simulink subsystem "ConfiguredSimulinkPlantModels"  (R2022b)
settings: Solver=VariableStepAuto  StartTime=0.0  StopTime=10.0  RelTol=1e-3
undefined symbols (not defined in the file): OCV, OCV_SoC, PlntTrnsfrCaseAxlSpdLock, PlntTrnsfrCaseTrqSplitRatio, soc_init
settings Model: Creator=The MathWorks, Inc.  LastModifiedBy=Thomas

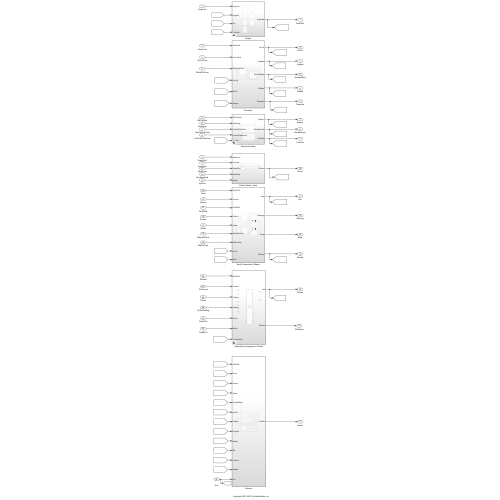
[thumbnail: Simulink's stored preview of the top-level diagram]
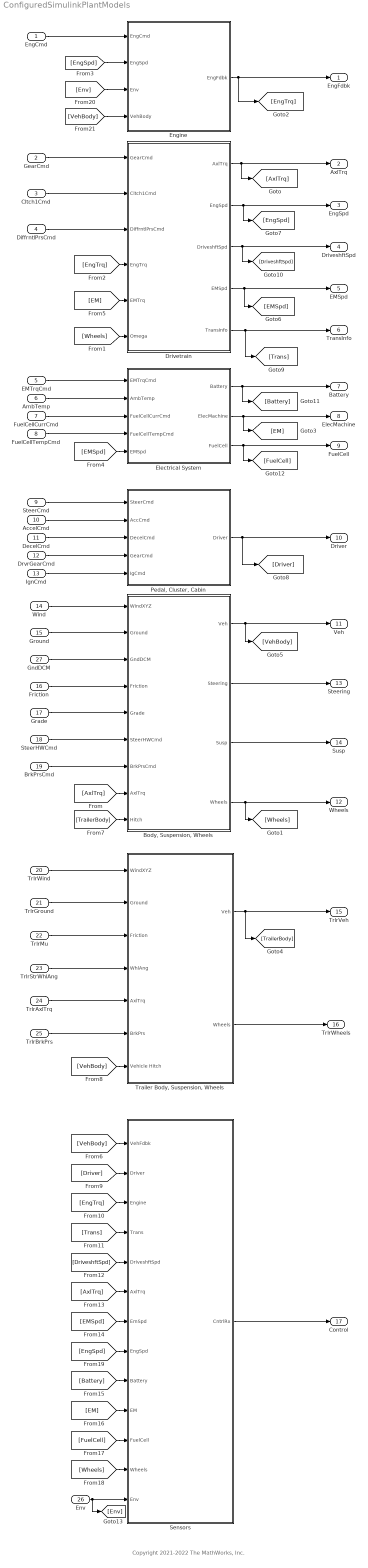
== system ConfiguredSimulinkPlantModels ==
  note: Copyright 2021-2022 The MathWorks, Inc.
  EngCmd : Inport
  GearCmd : Inport  Port=2
  Cltch1Cmd : Inport  Port=3
  DiffrntlPrsCmd : Inport  Port=4
  EMTrqCmd : Inport  Port=5
  AmbTemp : Inport  Port=6
  FuelCellCurrCmd : Inport  Port=7
  FuelCellTempCmd : Inport  Port=8
  SteerCmd : Inport  Port=9
  AccelCmd : Inport  Port=10
  DecelCmd : Inport  Port=11
  DrvrGearCmd : Inport  Port=12
  IgnCmd : Inport  Port=13
  Wind : Inport  Port=14
  Ground : Inport  Port=15
  Friction : Inport  Port=16
  Grade : Inport  Port=17
  SteerHWCmd : Inport  Port=18
  BrkPrsCmd : Inport  Port=19
  TrlrWind : Inport  Port=20
  TrlrGround : Inport  Port=21
  TrlrMu : Inport  Port=22
  TrlrStrWhlAng : Inport  Port=23
  TrlrAxlTrq : Inport  Port=24
  TrlrBrkPrs : Inport  Port=25
  " Env" : Inport  Port=26
  GndDCM : Inport  Port=27
  "Body, Suspension, Wheels" : Subsystem  VariantControl=Lateral Vehicle Dynamics
  Drivetrain : Subsystem
  Electrical System : Subsystem  Variant=on  VariantControlMode=label  VariantControl=Choice  LabelModeActiveChoice=Electrical System 1EM
  Engine : Subsystem  Variant=on  VariantControlMode=label  LabelModeActiveChoice=No Engine
  "Pedal, Cluster, Cabin" : Subsystem
  Sensors : Subsystem
  "Trailer Body, Suspension, Wheels" : Subsystem  Variant=on  VariantControlMode=label  LabelModeActiveChoice=No Trailer
  EngFdbk : Outport
  AxlTrq : Outport  Port=2
  EngSpd : Outport  Port=3
  DriveshftSpd : Outport  Port=4
  EMSpd : Outport  Port=5
  TransInfo : Outport  Port=6
  Battery : Outport  Port=7
  ElecMachine : Outport  Port=8
  FuelCell : Outport  Port=9
  Driver : Outport  Port=10
  Veh : Outport  Port=11
  Wheels : Outport  Port=12
  Steering : Outport  Port=13
  Susp : Outport  Port=14
  TrlrVeh : Outport  Port=15
  TrlrWheels : Outport  Port=16
  Control : Outport  Port=17
  wires:
  [EngSpd] -> Sensors/8(EngSpd)
  Cltch1Cmd/1 -> Drivetrain/2(Cltch1Cmd)
  FuelCellTempCmd/1 -> Electrical System/4(FuelCellTempCmd)
  "Body, Suspension, Wheels"/1(Veh) -> Veh/1, [VehBody]
  Electrical System/3(FuelCell) -> FuelCell/1, [FuelCell]
  [EngSpd] -> Engine/2(EngSpd)
  "Body, Suspension, Wheels"/3(Susp) -> Susp/1
  Grade/1 -> "Body, Suspension, Wheels"/5(Grade)
  [VehBody] -> Sensors/1(VehFdbk)
  SteerHWCmd/1 -> "Body, Suspension, Wheels"/6(SteerHWCmd)
  "Pedal, Cluster, Cabin"/1(Driver) -> Driver/1, [Driver]
  " Env"/1 -> Sensors/13(Env), [Env]
  [Driver] -> Sensors/2(Driver)
  AccelCmd/1 -> "Pedal, Cluster, Cabin"/2(AccCmd)
  [VehBody] -> Engine/4(VehBody)
  Drivetrain/3(DriveshftSpd) -> DriveshftSpd/1, [DriveshftSpd]
  [Wheels] -> Drivetrain/6(Omega)
  [EngTrq] -> Drivetrain/4(EngTrq)
  [Env] -> Engine/3(Env)
  IgnCmd/1 -> "Pedal, Cluster, Cabin"/5(IgCmd)
  TrlrGround/1 -> "Trailer Body, Suspension, Wheels"/2(Ground)
  [Battery] -> Sensors/9(Battery)
  [FuelCell] -> Sensors/11(FuelCell)
  [EM] -> Sensors/10(EM)
  [DriveshftSpd] -> Sensors/5(DriveshftSpd)
  [AxlTrq] -> Sensors/6(AxlTrq)
  DecelCmd/1 -> "Pedal, Cluster, Cabin"/3(DecelCmd)
  Drivetrain/4(EMSpd) -> EMSpd/1, [EMSpd]
  "Body, Suspension, Wheels"/4(Wheels) -> [Wheels], Wheels/1
  GearCmd/1 -> Drivetrain/1(GearCmd)
  SteerCmd/1 -> "Pedal, Cluster, Cabin"/1(SteerCmd)
  DrvrGearCmd/1 -> "Pedal, Cluster, Cabin"/4(GearCmd)
  [VehBody] -> "Trailer Body, Suspension, Wheels"/7(Vehicle Hitch)
  Friction/1 -> "Body, Suspension, Wheels"/4(Friction)
  EMTrqCmd/1 -> Electrical System/1(EMTrqCmd)
  GndDCM/1 -> "Body, Suspension, Wheels"/3(GndDCM)
  Sensors/1(CntrlRx) -> Control/1
  [EngTrq] -> Sensors/3(Engine)
  Electrical System/2(ElecMachine) -> ElecMachine/1, [EM]
  Drivetrain/2(EngSpd) -> EngSpd/1, [EngSpd]
  [Trans] -> Sensors/4(Trans)
  Wind/1 -> "Body, Suspension, Wheels"/1(WindXYZ)
  "Trailer Body, Suspension, Wheels"/1(Veh) -> TrlrVeh/1, [TrailerBody]
  TrlrBrkPrs/1 -> "Trailer Body, Suspension, Wheels"/6(BrkPrs)
  TrlrWind/1 -> "Trailer Body, Suspension, Wheels"/1(WindXYZ)
  DiffrntlPrsCmd/1 -> Drivetrain/3(DiffrntlPrsCmd)
  Drivetrain/1(AxlTrq) -> AxlTrq/1, [AxlTrq]
  BrkPrsCmd/1 -> "Body, Suspension, Wheels"/7(BrkPrsCmd)
  TrlrStrWhlAng/1 -> "Trailer Body, Suspension, Wheels"/4(WhlAng)
  TrlrMu/1 -> "Trailer Body, Suspension, Wheels"/3(Friction)
  EngCmd/1 -> Engine/1(EngCmd)
  [EM] -> Drivetrain/5(EMTrq)
  "Body, Suspension, Wheels"/2(Steering) -> Steering/1
  Engine/1(EngFdbk) -> EngFdbk/1, [EngTrq]
  Ground/1 -> "Body, Suspension, Wheels"/2(Ground)
  TrlrAxlTrq/1 -> "Trailer Body, Suspension, Wheels"/5(AxlTrq)
  [AxlTrq] -> "Body, Suspension, Wheels"/8(AxlTrq)
  [TrailerBody] -> "Body, Suspension, Wheels"/9(Hitch)
  AmbTemp/1 -> Electrical System/2(AmbTemp)
  Drivetrain/5(TransInfo) -> TransInfo/1, [Trans]
  Electrical System/1(Battery) -> Battery/1, [Battery]
  "Trailer Body, Suspension, Wheels"/2(Wheels) -> TrlrWheels/1
  [Wheels] -> Sensors/12(Wheels)
  [EMSpd] -> Sensors/7(EmSpd)
  FuelCellCurrCmd/1 -> Electrical System/3(FuelCellCurrCmd)
  [EMSpd] -> Electrical System/5(EMSpd)

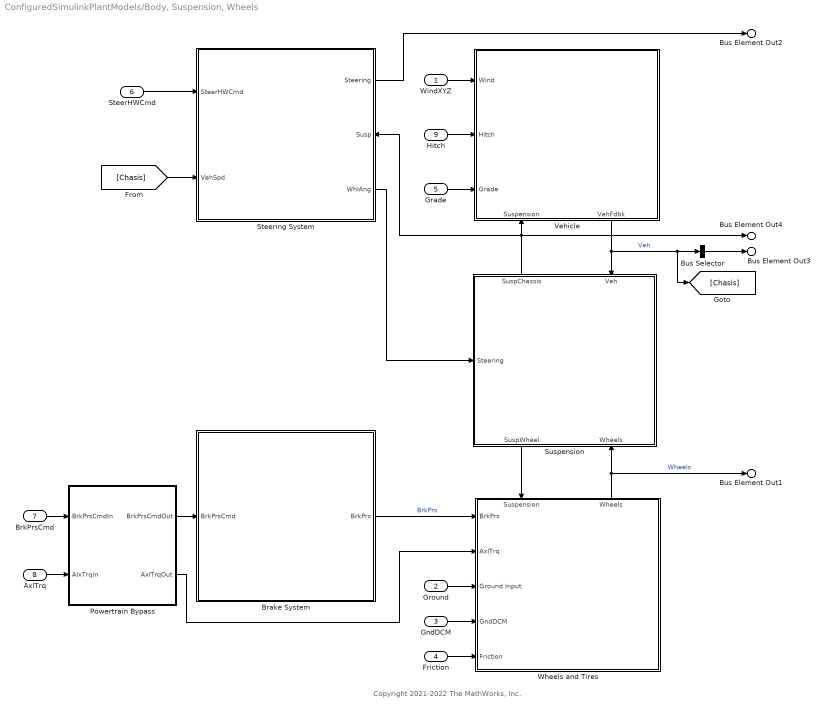
== system ConfiguredSimulinkPlantModels/Body, Suspension, Wheels ==
  note: Copyright 2021-2022 The MathWorks, Inc.
  WindXYZ : Inport  Unit=m/s  PortDimensions=3
  Ground : Inport  Port=2  Unit=m  PortDimensions=4
  GndDCM : Inport  Port=3
  Friction : Inport  Port=4  Unit=1  PortDimensions=4
  Grade : Inport  Port=5
  SteerHWCmd : Inport  Port=6  Unit=rad
  BrkPrsCmd : Inport  Port=7  PortDimensions=4
  AxlTrq : Inport  Port=8  Unit=N*m  PortDimensions=4
  Hitch : Inport  Port=9
  Brake System : Subsystem  Variant=on  VariantControlMode=label  VariantControl=Choice  LabelModeActiveChoice=BrakingHydraulics
      mask Display: disp('Brake System');
  Bus Selector : BusSelector  OutputSignals=InertFrm,BdyFrm  OutputAsBus=on
  Powertrain Bypass : Subsystem  Variant=on  VariantControlMode=label  VariantControl=Choice  LabelModeActiveChoice=Pass Through
  Steering System : Subsystem  Variant=on  VariantControlMode=label  VariantControl=0  LabelModeActiveChoice=No Steering
      settings: PortSchema="{\"entries\":[{\"content\":{\"sides\":[{\"content\":{\"connectorIds\":[\"In1\",\"In2\"]},\"type\":\"ConnectorPlacement.EquallySpacedRectSide\",\"uuid\":\"f4eae9a1-ee72-4894-9c3f-d81ee40fba89\"},{\"content\":{\"connectorIds\":[\"Out1\",\"In3\",\"Out2\"],\"side\":\"RIGHT\"},\"type\":\"ConnectorPlacement.EquallySpacedRectSide\",\"uuid\":\"c62a78d9-dc5d-4f96-a554-c82d7fa22a9e\"},{\"content\":{\"connectorIds\":[],\"side\":\"TOP\"},\"type\":\"ConnectorPlacement.EquallySpacedRectSide\",\"uuid\":\"38f3851a-1d1e-4a2b-8c09-8e5c8dcc7723\"}]},\"type\":\"ConnectorPlacement.EquallySpacedConnector\",\"uuid\":\"9f269846-92fa-4948-bc2b-71154f41fdde\"}],\"packageUris\":[\"http://schema.mathworks.com/mf0/Connector/R2020b\"],\"version\":\"1.0\"}"
      mask Display: disp('Steering System');
  Suspension : Subsystem  Variant=on  VariantControlMode=label  VariantControl=Choice  LabelModeActiveChoice=No Suspension
      settings: PortSchema="{\"entries\":[{\"content\":{\"sides\":[{\"content\":{\"connectorIds\":[\"In1\"]},\"type\":\"ConnectorPlacement.EquallySpacedRectSide\",\"uuid\":\"0a9265e3-f55e-4b74-9b74-681dc9522591\"},{\"content\":{\"connectorIds\":[],\"side\":\"RIGHT\"},\"type\":\"ConnectorPlacement.EquallySpacedRectSide\",\"uuid\":\"92df639a-7bc2-4e90-97ea-0cb216e2f16a\"},{\"content\":{\"connectorIds\":[\"Out2\",\"In2\"],\"side\":\"TOP\"},\"type\":\"ConnectorPlacement.EquallySpacedRectSide\",\"uuid\":\"2064b6cb-c7a8-4cfb-82de-a07750d990cb\"},{\"content\":{\"connectorIds\":[\"Out1\",\"In3\"],\"side\":\"BOTTOM\"},\"type\":\"ConnectorPlacement.EquallySpacedRectSide\",\"uuid\":\"169bd4e6-c3fe-4e36-acea-c25875014463\"}]},\"type\":\"ConnectorPlacement.EquallySpacedConnector\",\"uuid\":\"e0b50182-0637-4594-80e7-4ddd0df85797\"}],\"packageUris\":[\"http://schema.mathworks.com/mf0/Connector/R2020b\"],\"version\":\"1.0\"}"
      mask Display: disp('Suspension');
  Vehicle : Subsystem  Variant=on  VariantControlMode=label  VariantControl=Choice  LabelModeActiveChoice=Vehicle Body 3DOF Longitudinal
      settings: PortSchema="{\"entries\":[{\"content\":{\"sides\":[{\"content\":{\"connectorIds\":[\"In1\",\"In2\",\"In3\"]},\"type\":\"ConnectorPlacement.EquallySpacedRectSide\",\"uuid\":\"0a9265e3-f55e-4b74-9b74-681dc9522591\"},{\"content\":{\"connectorIds\":[],\"side\":\"RIGHT\"},\"type\":\"ConnectorPlacement.EquallySpacedRectSide\",\"uuid\":\"92df639a-7bc2-4e90-97ea-0cb216e2f16a\"},{\"content\":{\"connectorIds\":[],\"side\":\"TOP\"},\"type\":\"ConnectorPlacement.EquallySpacedRectSide\",\"uuid\":\"2064b6cb-c7a8-4cfb-82de-a07750d990cb\"},{\"content\":{\"connectorIds\":[\"In4\",\"Out1\"],\"side\":\"BOTTOM\"},\"type\":\"ConnectorPlacement.EquallySpacedRectSide\",\"uuid\":\"2b34afca-0a88-43db-924f-6476183b84bd\"}]},\"type\":\"ConnectorPlacement.EquallySpacedConnector\",\"uuid\":\"e0b50182-0637-4594-80e7-4ddd0df85797\"}],\"packageUris\":[\"http://schema.mathworks.com/mf0/Connector/R2020b\"],\"version\":\"1.0\"}"
      mask Display: disp('Vehicle');
  Wheels and Tires : Subsystem  Variant=on  VariantControlMode=label  VariantControl=Choice  LabelModeActiveChoice=MF Tires Longitudinal
      settings: PortSchema="{\"entries\":[{\"content\":{\"sides\":[{\"content\":{\"connectorIds\":[\"In1\",\"In2\",\"In3\",\"In4\",\"In5\"]},\"type\":\"ConnectorPlacement.EquallySpacedRectSide\",\"uuid\":\"fdb4d4cd-d0c0-42d9-b073-775af31e96a1\"},{\"content\":{\"connectorIds\":[],\"side\":\"RIGHT\"},\"type\":\"ConnectorPlacement.EquallySpacedRectSide\",\"uuid\":\"04106ddf-9917-4cd4-b177-ae763d642686\"},{\"content\":{\"connectorIds\":[\"In6\",\"Out1\"],\"side\":\"TOP\"},\"type\":\"ConnectorPlacement.EquallySpacedRectSide\",\"uuid\":\"568bf95c-0e25-4c45-a134-c198357b75be\"}]},\"type\":\"ConnectorPlacement.EquallySpacedConnector\",\"uuid\":\"4f44df5e-0d14-43ea-934e-2abe86546e95\"}],\"packageUris\":[\"http://schema.mathworks.com/mf0/Connector/R2020b\"],\"version\":\"1.0\"}"
      mask Display: disp('Wheels and Tires');
  Bus Element Out3 : Outport  PortName=Veh
  Bus Element Out2 : Outport  Port=2  PortName=Steering
  Bus Element Out4 : Outport  Port=3  PortName=Susp
  Bus Element Out1 : Outport  Port=4  PortName=Wheels
  wires:
  GndDCM/1 -> Wheels and Tires/4(GndDCM)
  Friction/1 -> Wheels and Tires/5(Friction)
  Powertrain Bypass/2(AxlTrqOut) -> Wheels and Tires/2(AxlTrq)
  Ground/1 -> Wheels and Tires/3(Ground Input)
  Grade/1 -> Vehicle/3(Grade)
  Wheels and Tires/1(Wheels) -> Suspension/3(Wheels), Bus Element Out1/1  "Wheels"
  Suspension/1(SuspWheel) -> Wheels and Tires/6(Suspension)
  Brake System/1(BrkPrs) -> Wheels and Tires/1(BrkPrs)  "BrkPrs"
  Vehicle/1(VehFdbk) -> Suspension/2(Veh), [Chasis], Bus Selector/1  "Veh"
  Hitch/1 -> Vehicle/2(Hitch)
  WindXYZ/1 -> Vehicle/1(Wind)
  Suspension/2(SuspChassis) -> Bus Element Out4/1, Vehicle/4(Suspension), Steering System/3(Susp)
  Steering System/2(WhlAng) -> Suspension/1(Steering)
  BrkPrsCmd/1 -> Powertrain Bypass/1(BrkPrsCmdIn)
  Bus Selector/1 -> Bus Element Out3/1
  [Chasis] -> Steering System/2(VehSpd)
  SteerHWCmd/1 -> Steering System/1(SteerHWCmd)
  Steering System/1(Steering) -> Bus Element Out2/1
  Powertrain Bypass/1(BrkPrsCmdOut) -> Brake System/1(BrkPrsCmd)
  AxlTrq/1 -> Powertrain Bypass/2(AlxTrqIn)

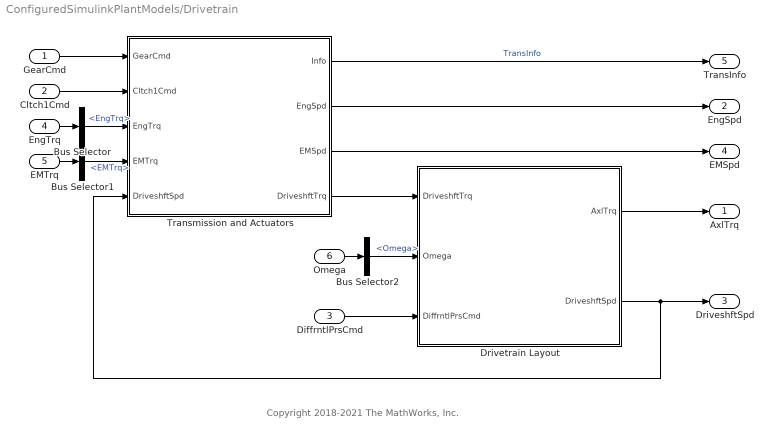
== system ConfiguredSimulinkPlantModels/Drivetrain ==
  note: Copyright 2018-2021 The MathWorks, Inc.
  GearCmd : Inport
  Cltch1Cmd : Inport  Port=2
  DiffrntlPrsCmd : Inport  Port=3
  EngTrq : Inport  Port=4
  EMTrq : Inport  Port=5
  Omega : Inport  Port=6
  Bus Selector : BusSelector  OutputSignals=EngTrq
  Bus Selector1 : BusSelector  OutputSignals=EMTrq
  Bus Selector2 : BusSelector  OutputSignals=Wheels.Omega
  Drivetrain Layout : Subsystem  VariantControl=New
  Transmission and Actuators : Subsystem  Variant=on  VariantControlMode=label  LabelModeActiveChoice=Electric Vehicle 1EM
  AxlTrq : Outport  VectorParamsAs1DForOutWhenUnconnected=off
  EngSpd : Outport  Port=2  Unit=rad/s  VectorParamsAs1DForOutWhenUnconnected=off
  DriveshftSpd : Outport  Port=3  VectorParamsAs1DForOutWhenUnconnected=off
  EMSpd : Outport  Port=4  Unit=rad/s  VectorParamsAs1DForOutWhenUnconnected=off
  TransInfo : Outport  Port=5  VectorParamsAs1DForOutWhenUnconnected=off
  wires:
  Transmission and Actuators/1(Info) -> TransInfo/1  "TransInfo"
  DiffrntlPrsCmd/1 -> Drivetrain Layout/3(DiffrntlPrsCmd)
  Cltch1Cmd/1 -> Transmission and Actuators/2(Cltch1Cmd)
  Drivetrain Layout/2(DriveshftSpd) -> DriveshftSpd/1, Transmission and Actuators/5(DriveshftSpd)
  GearCmd/1 -> Transmission and Actuators/1(GearCmd)
  Drivetrain Layout/1(AxlTrq) -> AxlTrq/1
  Transmission and Actuators/2(EngSpd) -> EngSpd/1
  Transmission and Actuators/3(EMSpd) -> EMSpd/1
  Transmission and Actuators/4(DriveshftTrq) -> Drivetrain Layout/1(DriveshftTrq)
  EngTrq/1 -> Bus Selector/1
  Bus Selector/1 -> Transmission and Actuators/3(EngTrq)  "<EngTrq>"
  EMTrq/1 -> Bus Selector1/1
  Bus Selector1/1 -> Transmission and Actuators/4(EMTrq)  "<EMTrq>"
  Omega/1 -> Bus Selector2/1
  Bus Selector2/1 -> Drivetrain Layout/2(Omega)  "<Omega>"

== system ConfiguredSimulinkPlantModels/Electrical System ==
  EMTrqCmd : Inport
  AmbTemp : Inport  Port=2
  FuelCellCurrCmd : Inport  Port=3
  FuelCellTempCmd : Inport  Port=4
  EMSpd : Inport  Port=5
  Electrical System 1EM : Subsystem  VariantControl=Electrical System 1EM
  Battery : Outport
  ElecMachine : Outport  Port=2
  FuelCell : Outport  Port=3

== system ConfiguredSimulinkPlantModels/Engine ==
  EngCmd : Inport
  EngSpd : Inport  Port=2
  Env : Inport  Port=3
  VehBody : Inport  Port=4
  No Engine : Subsystem  VariantControl=No Engine
  EngFdbk : Outport  VectorParamsAs1DForOutWhenUnconnected=off

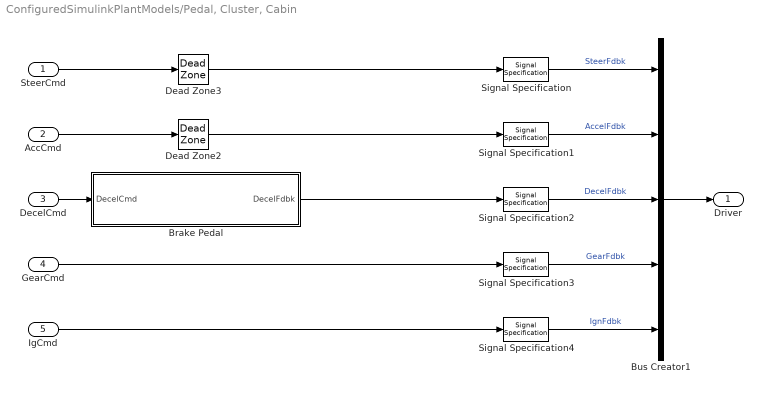
== system ConfiguredSimulinkPlantModels/Pedal, Cluster, Cabin ==
  SteerCmd : Inport
  AccCmd : Inport  Port=2
  DecelCmd : Inport  Port=3
  GearCmd : Inport  Port=4
  IgCmd : Inport  Port=5
  Brake Pedal : Subsystem
  Bus Creator1 : BusCreator  Inputs=5
  Dead Zone2 : DeadZone  LowerValue=0  UpperValue=.01  ZeroCross=off
  Dead Zone3 : DeadZone  LowerValue=-.01  UpperValue=.01  ZeroCross=off
  Signal Specification : SignalSpecification  Unit=rad
  Signal Specification{1..4} (4 alike) : SignalSpecification  Unit=1
  Driver : Outport
  wires:
  Dead Zone3/1 -> Signal Specification/1
  Signal Specification1/1 -> Bus Creator1/2  "AccelFdbk"
  Signal Specification4/1 -> Bus Creator1/5  "IgnFdbk"
  Brake Pedal/1(DecelFdbk) -> Signal Specification2/1
  Signal Specification/1 -> Bus Creator1/1  "SteerFdbk"
  Signal Specification2/1 -> Bus Creator1/3  "DecelFdbk"
  GearCmd/1 -> Signal Specification3/1
  Bus Creator1/1 -> Driver/1
  IgCmd/1 -> Signal Specification4/1
  Signal Specification3/1 -> Bus Creator1/4  "GearFdbk"
  Dead Zone2/1 -> Signal Specification1/1
  SteerCmd/1 -> Dead Zone3/1
  AccCmd/1 -> Dead Zone2/1
  DecelCmd/1 -> Brake Pedal/1(DecelCmd)

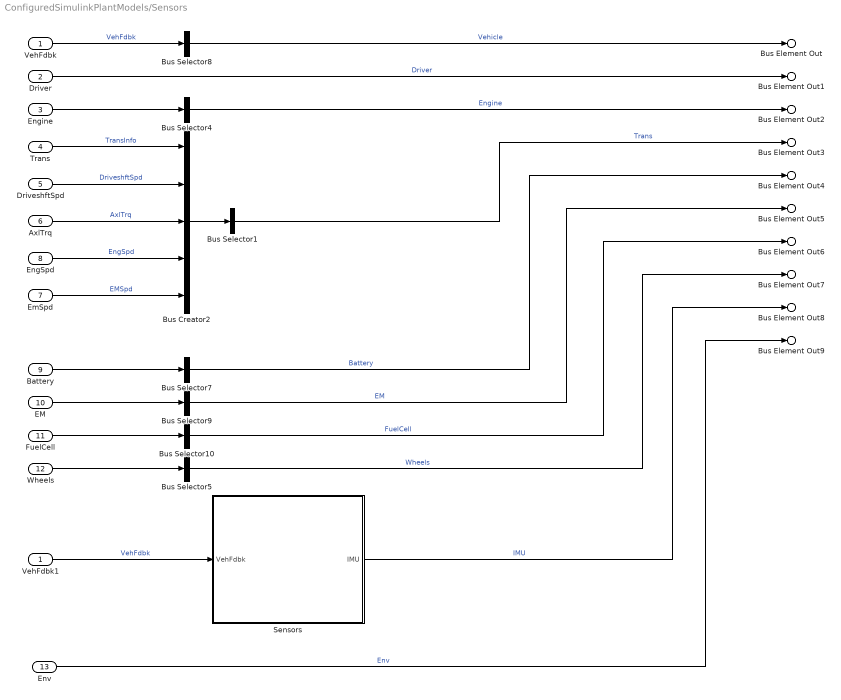
== system ConfiguredSimulinkPlantModels/Sensors ==
  VehFdbk : Inport
  Driver : Inport  Port=2
  Engine : Inport  Port=3
  Trans : Inport  Port=4
  DriveshftSpd : Inport  Port=5
  AxlTrq : Inport  Port=6
  EmSpd : Inport  Port=7
  EngSpd : Inport  Port=8
  Battery : Inport  Port=9
  EM : Inport  Port=10
  FuelCell : Inport  Port=11
  Wheels : Inport  Port=12
  Env : Inport  Port=13
  Bus Creator2 : BusCreator  Inputs=5
  Bus Selector1 : BusSelector  OutputSignals=TransInfo.Cltch1State,TransInfo.Cltch2State,DriveshftSpd,AxlTrq,EngSpd,EMSpd,TransInfo.TransInfo.Trans.TransGear  OutputAsBus=on
  Bus Selector10 : BusSelector  OutputSignals=FuelCellVolt,FuelCellCurr,H2Flw  OutputAsBus=on
  Bus Selector4 : BusSelector  OutputSignals=EngTrq,Map,Mat,ThrPosPct,WgAreaPct,IntkCamPhase,ExhCamPhase,TurboRackPos,EgrVlvAreaPct,VarCompRatioPos,IntkVlvLift,VarIntkRunLen,Afr,IntkSwirlVlvPos,TurboSpd,Iat,Ect,EgrVlvDeltaPrs,EgrVlvInTemp  OutputAsBus=on
  Bus Selector5 : BusSelector  OutputSignals=Wheels.BrkPrs,Wheels.Kappa,Wheels.Alpha,Wheels.Omega  OutputAsBus=on
  Bus Selector7 : BusSelector  OutputSignals=BattSoc,BattVolt,BattCurr,BattPwr,BMSSensors  OutputAsBus=on
  Bus Selector8 : BusSelector  OutputSignals=BdyFrm.Cg.Vel.xdot  OutputAsBus=on
  Bus Selector9 : BusSelector  OutputSignals=EMTrq,EMPwrElec  OutputAsBus=on
  Sensors : Subsystem  Variant=on  VariantControlMode=label  VariantControl=Choice  LabelModeActiveChoice=No IMU Sensor
  VehFdbk1 : InportShadow
  Bus Element Out : Outport  PortName=CntrlRx  Element=Vehicle
  Bus Element Out1 : Outport  PortName=CntrlRx  Element=Driver
  Bus Element Out2 : Outport  PortName=CntrlRx  Element=Engine
  Bus Element Out3 : Outport  PortName=CntrlRx  Element=Trans
  Bus Element Out4 : Outport  PortName=CntrlRx  Element=Battery
  Bus Element Out5 : Outport  PortName=CntrlRx  Element=EM
  Bus Element Out6 : Outport  PortName=CntrlRx  Element=FuelCell
  Bus Element Out7 : Outport  PortName=CntrlRx  Element=Wheels
  Bus Element Out8 : Outport  PortName=CntrlRx  Element=IMU
  Bus Element Out9 : Outport  PortName=CntrlRx  Element=Env
  wires:
  Bus Selector1/1 -> Bus Element Out3/1  "Trans"
  Bus Creator2/1 -> Bus Selector1/1
  Trans/1 -> Bus Creator2/1  "TransInfo"
  EngSpd/1 -> Bus Creator2/4  "EngSpd"
  Env/1 -> Bus Element Out9/1  "Env"
  Driver/1 -> Bus Element Out1/1  "Driver"
  Sensors/1(IMU) -> Bus Element Out8/1  "IMU"
  VehFdbk1/1 -> Sensors/1(VehFdbk)  "VehFdbk"
  Wheels/1 -> Bus Selector5/1
  FuelCell/1 -> Bus Selector10/1
  EM/1 -> Bus Selector9/1
  Battery/1 -> Bus Selector7/1
  EmSpd/1 -> Bus Creator2/5  "EMSpd"
  AxlTrq/1 -> Bus Creator2/3  "AxlTrq"
  DriveshftSpd/1 -> Bus Creator2/2  "DriveshftSpd"
  Engine/1 -> Bus Selector4/1
  VehFdbk/1 -> Bus Selector8/1  "VehFdbk"
  Bus Selector4/1 -> Bus Element Out2/1  "Engine"
  Bus Selector10/1 -> Bus Element Out6/1  "FuelCell"
  Bus Selector9/1 -> Bus Element Out5/1  "EM"
  Bus Selector8/1 -> Bus Element Out/1  "Vehicle"
  Bus Selector7/1 -> Bus Element Out4/1  "Battery"
  Bus Selector5/1 -> Bus Element Out7/1  "Wheels"

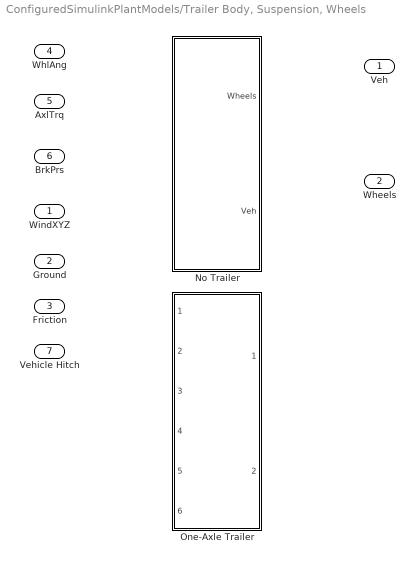
== system ConfiguredSimulinkPlantModels/Trailer Body, Suspension, Wheels ==
  WindXYZ : Inport
  Ground : Inport  Port=2
  Friction : Inport  Port=3
  WhlAng : Inport  Port=4
  AxlTrq : Inport  Port=5
  BrkPrs : Inport  Port=6
  Vehicle Hitch : Inport  Port=7
  No Trailer : Subsystem  VariantControl=No Trailer
  One-Axle Trailer : Subsystem  VariantControl=One-Axle Trailer  ReferencedSubsystem=OneAxleTrailer
  Veh : Outport  VectorParamsAs1DForOutWhenUnconnected=off
  Wheels : Outport  Port=2  VectorParamsAs1DForOutWhenUnconnected=off

== system ConfiguredSimulinkPlantModels/Body, Suspension, Wheels/Brake System ==
  BrkPrsCmd : Inport
  BrakingHydraulics : Subsystem  VariantControl=BrakingHydraulics  ReferencedSubsystem=BrakingHydraulics
  BrkPrs : Outport

== system ConfiguredSimulinkPlantModels/Body, Suspension, Wheels/Powertrain Bypass ==
  BrkPrsCmdIn : Inport
  AlxTrqIn : Inport  Port=2
  External Signal Source : Subsystem  VariantControl=External Signal Source
  Pass Through : Subsystem  VariantControl=Pass Through
  BrkPrsCmdOut : Outport
  AxlTrqOut : Outport  Port=2

== system ConfiguredSimulinkPlantModels/Body, Suspension, Wheels/Steering System ==
  SteerHWCmd : Inport
  VehSpd : Inport  Port=2
  Susp : Inport  Port=3
  No Steering : Subsystem  VariantControl=No Steering  ReferencedSubsystem=NoSteering
  Steering : Outport
  WhlAng : Outport  Port=2  VectorParamsAs1DForOutWhenUnconnected=off

== system ConfiguredSimulinkPlantModels/Body, Suspension, Wheels/Suspension ==
  Steering : Inport
  Veh : Inport  Port=2
  Wheels : Inport  Port=3
  No Suspension : Subsystem  VariantControl=No Suspension  ReferencedSubsystem=NoSuspension
  SuspWheel : Outport
  SuspChassis : Outport  Port=2

== system ConfiguredSimulinkPlantModels/Body, Suspension, Wheels/Vehicle ==
  Wind : Inport
  Hitch : Inport  Port=2
  Grade : Inport  Port=3
  Suspension : Inport  Port=4
  Vehicle Body 3DOF Longitudinal : Subsystem  VariantControl=Vehicle Body 3DOF Longitudinal  ReferencedSubsystem=VehicleBody3DOFLongitudinal
  VehFdbk : Outport

== system ConfiguredSimulinkPlantModels/Body, Suspension, Wheels/Wheels and Tires ==
  BrkPrs : Inport
  AxlTrq : Inport  Port=2
  Ground Input : Inport  Port=3
  GndDCM : Inport  Port=4
  Friction : Inport  Port=5
  Suspension : Inport  Port=6
  MF Tires Longitudinal : Subsystem  VariantControl=MF Tires Longitudinal  ReferencedSubsystem=MFTiresLongitudinal
  Wheels : Outport

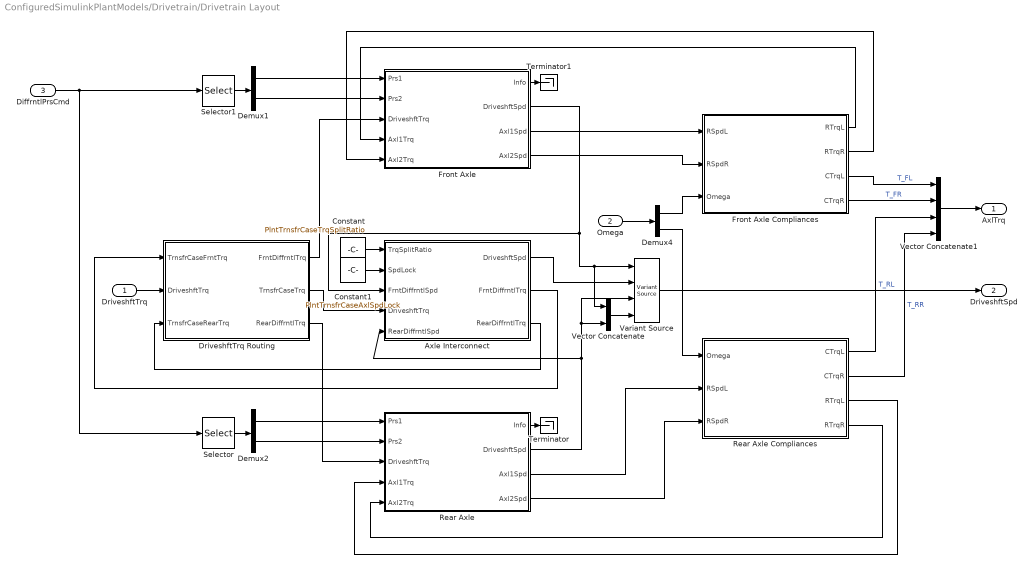
== system ConfiguredSimulinkPlantModels/Drivetrain/Drivetrain Layout ==
  DriveshftTrq : Inport
  Omega : Inport  Port=2
  DiffrntlPrsCmd : Inport  Port=3
  Axle Interconnect : Subsystem  Variant=on  VariantControlMode=label  VariantControl=Choice  LabelModeActiveChoice=No Interconnect
  Constant : Constant  Value=PlntTrnsfrCaseTrqSplitRatio  SampleTime=-1
  Constant1 : Constant  Value=PlntTrnsfrCaseAxlSpdLock  SampleTime=-1
  Demux1 : Demux  Outputs=2
  Demux2 : Demux  Outputs=2
  Demux4 : Demux  Outputs=2
  DriveshftTrq Routing : Subsystem  Variant=on  VariantControlMode=label  VariantControl=Choice  LabelModeActiveChoice=One Actuator FWD
  Front Axle : Subsystem  Variant=on  VariantControlMode=label  VariantControl=Choice  LabelModeActiveChoice=Open Differential
  Front Axle Compliances : Subsystem  Variant=on  VariantControlMode=label  VariantControl=Choice  LabelModeActiveChoice=Axle Compliances
  Rear Axle : Subsystem  Variant=on  VariantControlMode=label  VariantControl=Choice  LabelModeActiveChoice=No Differential
  Rear Axle Compliances : Subsystem  Variant=on  VariantControlMode=label  VariantControl=Choice  LabelModeActiveChoice=No Axle Compliances
  Selector : Selector  InputPortWidth=4  IndexOptions=Index vector (dialog)  Indices=[3 4]  OutputSizes=1
  Selector1 : Selector  InputPortWidth=4  IndexOptions=Index vector (dialog)  Indices=[1 2]  OutputSizes=1
  Terminator : Terminator
  Terminator1 : Terminator
  Variant Source : VariantSource  VariantControlMode=label  LabelModeActiveChoice=One Actuator FWD
  Vector Concatenate : Concatenate
  Vector Concatenate1 : Concatenate  NumInputs=4
  AxlTrq : Outport  VectorParamsAs1DForOutWhenUnconnected=off
  DriveshftSpd : Outport  Port=2  VectorParamsAs1DForOutWhenUnconnected=off
  wires:
  Selector/1 -> Demux2/1
  Demux2/1 -> Rear Axle/1(Prs1)
  Demux2/2 -> Rear Axle/2(Prs2)
  Demux1/2 -> Front Axle/2(Prs2)
  Demux1/1 -> Front Axle/1(Prs1)
  Selector1/1 -> Demux1/1
  Omega/1 -> Demux4/1
  Front Axle Compliances/1(RTrqL) -> Front Axle/4(Axl1Trq)
  Demux4/1 -> Front Axle Compliances/3(Omega)
  Front Axle Compliances/2(RTrqR) -> Front Axle/5(Axl2Trq)
  Front Axle/4(Axl2Spd) -> Front Axle Compliances/2(RSpdR)
  Front Axle/3(Axl1Spd) -> Front Axle Compliances/1(RSpdL)
  Front Axle Compliances/3(CTrqL) -> Vector Concatenate1/1  "T_FL"
  Front Axle Compliances/4(CTrqR) -> Vector Concatenate1/2  "T_FR"
  DiffrntlPrsCmd/1 -> Selector/1, Selector1/1
  Vector Concatenate1/1 -> AxlTrq/1
  Rear Axle/2(DriveshftSpd) -> Vector Concatenate/2, Variant Source/3, Axle Interconnect/5(RearDiffrntlSpd)
  Front Axle/2(DriveshftSpd) -> Axle Interconnect/3(FrntDiffrntlSpd), Variant Source/1, Vector Concatenate/1
  DriveshftTrq/1 -> DriveshftTrq Routing/2(DriveshftTrq)
  DriveshftTrq Routing/1(FrntDiffrntlTrq) -> Front Axle/3(DriveshftTrq)
  DriveshftTrq Routing/3(RearDiffrntlTrq) -> Rear Axle/3(DriveshftTrq)
  Rear Axle/1(Info) -> Terminator/1
  Front Axle/1(Info) -> Terminator1/1
  Variant Source/1 -> DriveshftSpd/1
  DriveshftTrq Routing/2(TrnsfrCaseTrq) -> Axle Interconnect/4(DriveshftTrq)
  Axle Interconnect/1(DriveshftSpd) -> Variant Source/2
  Axle Interconnect/2(FrntDiffrntlTrq) -> DriveshftTrq Routing/1(TrnsfrCaseFrntTrq)
  Axle Interconnect/3(RearDiffrntlTrq) -> DriveshftTrq Routing/3("TrnsfrCaseRearTrq ")
  Vector Concatenate/1 -> Variant Source/4
  Demux4/2 -> Rear Axle Compliances/1(Omega)
  Rear Axle/3(Axl1Spd) -> Rear Axle Compliances/2(RSpdL)
  Rear Axle/4(Axl2Spd) -> Rear Axle Compliances/3(RSpdR)
  Rear Axle Compliances/1(CTrqL) -> Vector Concatenate1/3  "T_RL"
  Rear Axle Compliances/2(CTrqR) -> Vector Concatenate1/4  "T_RR"
  Rear Axle Compliances/3(RTrqL) -> Rear Axle/4(Axl1Trq)
  Rear Axle Compliances/4(RTrqR) -> Rear Axle/5(Axl2Trq)
  Constant/1 -> Axle Interconnect/1(TrqSplitRatio)
  Constant1/1 -> Axle Interconnect/2(SpdLock)

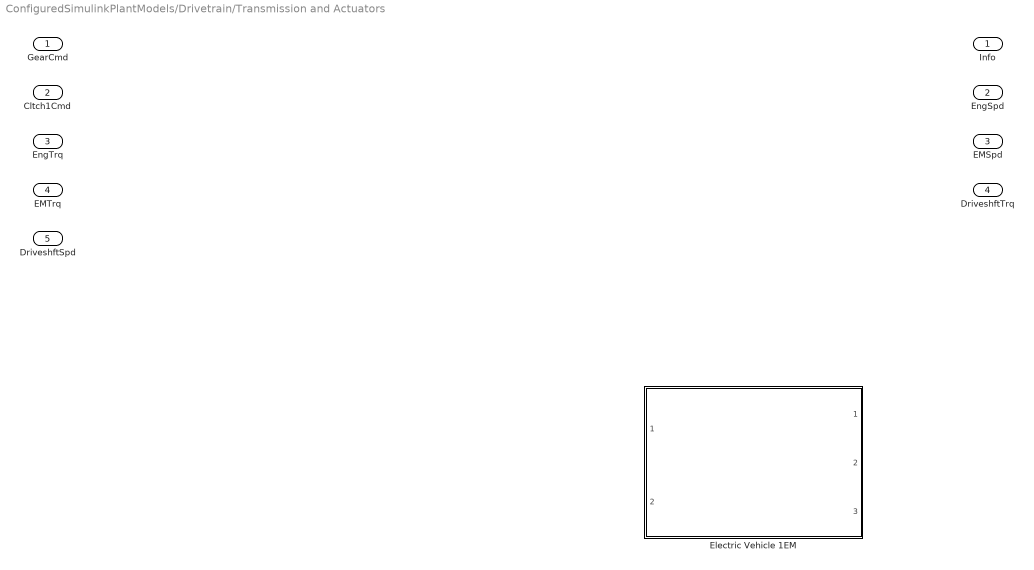
== system ConfiguredSimulinkPlantModels/Drivetrain/Transmission and Actuators ==
  GearCmd : Inport
  Cltch1Cmd : Inport  Port=2
  EngTrq : Inport  Port=3
  EMTrq : Inport  Port=4
  DriveshftSpd : Inport  Port=5
  Electric Vehicle 1EM : Subsystem  VariantControl=Electric Vehicle 1EM  ReferencedSubsystem=BEV1EM
  Info : Outport  VectorParamsAs1DForOutWhenUnconnected=off
  EngSpd : Outport  Port=2  VectorParamsAs1DForOutWhenUnconnected=off
  EMSpd : Outport  Port=3  VectorParamsAs1DForOutWhenUnconnected=off  BusOutputAsStruct=on
  DriveshftTrq : Outport  Port=4  VectorParamsAs1DForOutWhenUnconnected=off

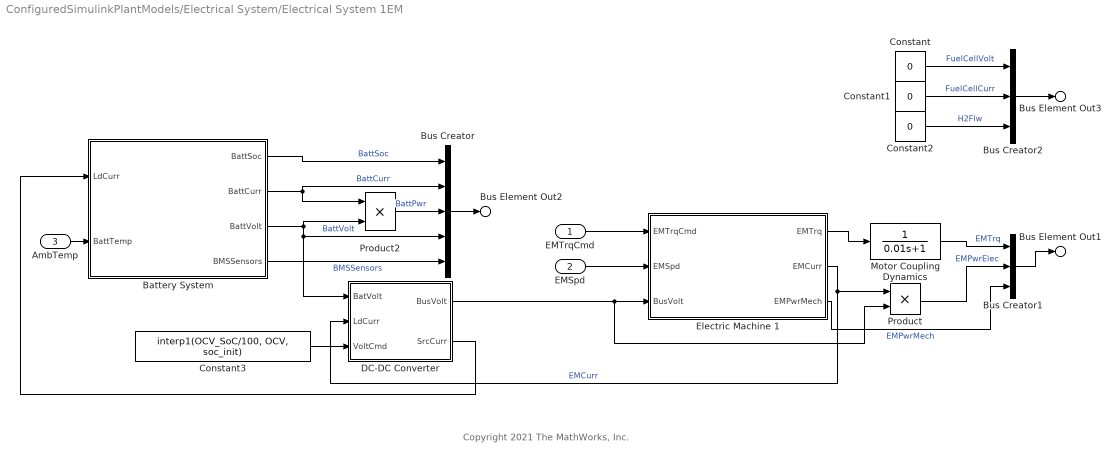
== system ConfiguredSimulinkPlantModels/Electrical System/Electrical System 1EM ==
  note: Copyright 2021 The MathWorks, Inc.
  EMTrqCmd : Inport
  EMSpd : Inport  Port=2
  AmbTemp : Inport  Port=3
  Battery System : Subsystem  Variant=on  VariantControlMode=label  LabelModeActiveChoice=Mapped Battery
  Bus Creator : BusCreator  Inputs=5
  Bus Creator1 : BusCreator  Inputs=3
  Bus Creator2 : BusCreator  Inputs=3
  Constant : Constant  Value=0  SampleTime=-1
  Constant1 : Constant  Value=0  SampleTime=-1
  Constant2 : Constant  Value=0  SampleTime=-1
  Constant3 : Constant  Value=interp1(OCV_SoC/100, OCV, soc_init)  SampleTime=-1
  DC-DC Converter : Subsystem  Variant=on  VariantControlMode=label  VariantControl=Choice  LabelModeActiveChoice=No DC-DC Converter
  Electric Machine 1 : Subsystem  Variant=on  VariantControlMode=label  LabelModeActiveChoice=Mapped EM
  Motor Coupling Dynamics : TransferFcn  Denominator=[0.01 1]
  Product : Product
  Product2 : Product
  Bus Element Out2 : Outport  PortName=Battery
  Bus Element Out1 : Outport  Port=2  PortName=ElecMachine
  Bus Element Out3 : Outport  Port=3  PortName=FuelCell
  wires:
  Electric Machine 1/3(EMPwrMech) -> Bus Creator1/3  "EMPwrMech"
  AmbTemp/1 -> Battery System/2(BattTemp)
  Battery System/2(BattCurr) -> Bus Creator/2, Product2/1  "BattCurr"
  EMTrqCmd/1 -> Electric Machine 1/1(EMTrqCmd)
  Electric Machine 1/2(EMCurr) -> DC-DC Converter/2(LdCurr), Product/1  "EMCurr"
  Battery System/1(BattSoc) -> Bus Creator/1  "BattSoc"
  EMSpd/1 -> Electric Machine 1/2(EMSpd)
  Battery System/3(BattVolt) -> DC-DC Converter/1(BatVolt), Bus Creator/4, Product2/2  "BattVolt"
  Product2/1 -> Bus Creator/3  "BattPwr"
  Bus Creator2/1 -> Bus Element Out3/1
  Product/1 -> Bus Creator1/2  "EMPwrElec"
  Bus Creator1/1 -> Bus Element Out1/1
  Motor Coupling Dynamics/1 -> Bus Creator1/1  "EMTrq"
  Constant/1 -> Bus Creator2/1  "FuelCellVolt"
  Electric Machine 1/1(EMTrq) -> Motor Coupling Dynamics/1
  Constant1/1 -> Bus Creator2/2  "FuelCellCurr"
  Bus Creator/1 -> Bus Element Out2/1
  Constant2/1 -> Bus Creator2/3  "H2Flw"
  DC-DC Converter/1(BusVolt) -> Product/2, Electric Machine 1/3(BusVolt)
  DC-DC Converter/2(SrcCurr) -> Battery System/1(LdCurr)
  Constant3/1 -> DC-DC Converter/3(VoltCmd)
  Battery System/4(BMSSensors) -> Bus Creator/5  "BMSSensors"

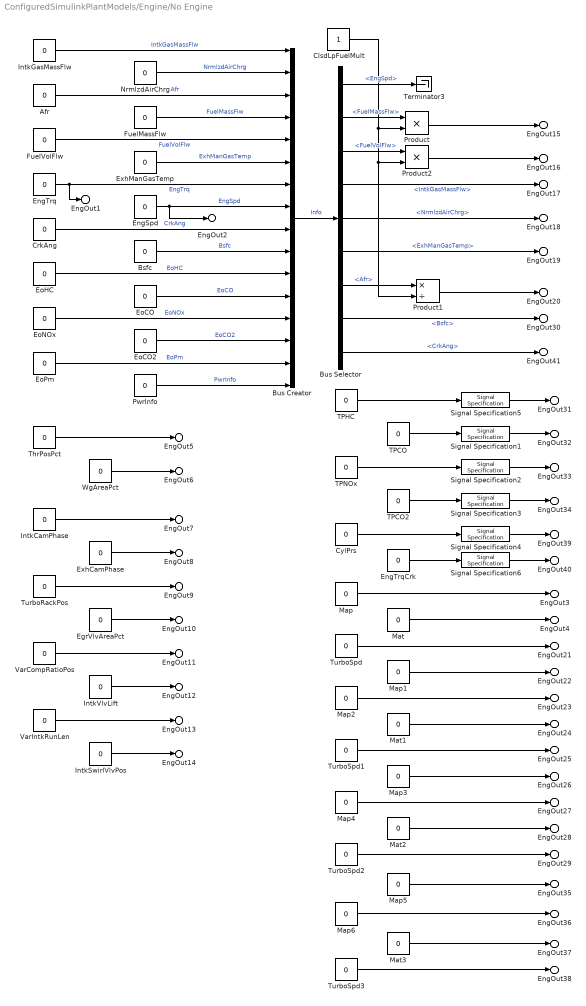
== system ConfiguredSimulinkPlantModels/Engine/No Engine ==
  Afr : Constant  Value=0
  Bsfc : Constant  Value=0
  Bus Creator : BusCreator  Inputs=16
  Bus Selector : BusSelector  OutputSignals=EngSpd,FuelMassFlw,FuelVolFlw,IntkGasMassFlw,NrmlzdAirChrg,ExhManGasTemp,Afr,Bsfc,CrkAng
  ClsdLpFuelMult : Constant
  CrkAng : Constant  Value=0
  CylPrs : Constant  Value=0
  EgrVlvAreaPct : Constant  Value=0
  EngSpd : Constant  Value=0
  EngTrq : Constant  Value=0
  EngTrqCrk : Constant  Value=0
  EoCO : Constant  Value=0
  EoCO2 : Constant  Value=0
  EoHC : Constant  Value=0
  EoNOx : Constant  Value=0
  EoPm : Constant  Value=0
  ExhCamPhase : Constant  Value=0
  ExhManGasTemp : Constant  Value=0
  FuelMassFlw : Constant  Value=0
  FuelVolFlw : Constant  Value=0
  IntkCamPhase : Constant  Value=0
  IntkGasMassFlw : Constant  Value=0
  IntkSwirlVlvPos : Constant  Value=0
  IntkVlvLift : Constant  Value=0
  Map{,1..6} (7 alike) : Constant  Value=0
  Mat{,1..3} (4 alike) : Constant  Value=0
  NrmlzdAirChrg : Constant  Value=0
  Product : Product
  Product1 : Product  Inputs=*/
  Product2 : Product
  PwrInfo : Constant  Value=0
  Signal Specification{1..3,5} (4 alike) : SignalSpecification  Unit=kg/s
  Signal Specification4 : SignalSpecification  Unit=Pa
  Signal Specification6 : SignalSpecification  Unit=N*m
  TPCO : Constant  Value=0
  TPCO2 : Constant  Value=0
  TPHC : Constant  Value=0
  TPNOx : Constant  Value=0
  Terminator3 : Terminator
  ThrPosPct : Constant  Value=0
  TurboRackPos : Constant  Value=0
  TurboSpd{,1..3} (4 alike) : Constant  Value=0
  VarCompRatioPos : Constant  Value=0
  VarIntkRunLen : Constant  Value=0
  WgAreaPct : Constant  Value=0
  EngOut1 : Outport  PortName=EngFdbk  Element=EngTrq
  EngOut2 : Outport  PortName=EngFdbk  Element=EngSpdOut
  EngOut3 : Outport  PortName=EngFdbk  Element=Map
  EngOut4 : Outport  PortName=EngFdbk  Element=Mat
  EngOut5 : Outport  PortName=EngFdbk  Element=ThrPosPct
  EngOut6 : Outport  PortName=EngFdbk  Element=WgAreaPct
  EngOut7 : Outport  PortName=EngFdbk  Element=IntkCamPhase
  EngOut8 : Outport  PortName=EngFdbk  Element=ExhCamPhase
  EngOut9 : Outport  PortName=EngFdbk  Element=TurboRackPos
  EngOut10 : Outport  PortName=EngFdbk  Element=EgrVlvAreaPct
  EngOut11 : Outport  PortName=EngFdbk  Element=VarCompRatioPos
  EngOut12 : Outport  PortName=EngFdbk  Element=IntkVlvLift
  EngOut13 : Outport  PortName=EngFdbk  Element=VarIntkRunLen
  EngOut14 : Outport  PortName=EngFdbk  Element=IntkSwirlVlvPos
  EngOut15 : Outport  PortName=EngFdbk  Element=FuelFlw
  EngOut16 : Outport  PortName=EngFdbk  Element=FuelVolFlw
  EngOut17 : Outport  PortName=EngFdbk  Element=IntkPortFlw
  EngOut18 : Outport  PortName=EngFdbk  Element=NormAirChrg
  EngOut19 : Outport  PortName=EngFdbk  Element=ExhManGasTemp
  EngOut20 : Outport  PortName=EngFdbk  Element=Afr
  EngOut21 : Outport  PortName=EngFdbk  Element=TurboSpd
  EngOut22 : Outport  PortName=EngFdbk  Element=TurbPrsRatio
  EngOut23 : Outport  PortName=EngFdbk  Element=CompPrsRatio
  EngOut24 : Outport  PortName=EngFdbk  Element=TurbTempOut
  EngOut25 : Outport  PortName=EngFdbk  Element=CompTempOut
  EngOut26 : Outport  PortName=EngFdbk  Element=EgrPct
  EngOut27 : Outport  PortName=EngFdbk  Element=EgrMassFlwRate
  EngOut28 : Outport  PortName=EngFdbk  Element=EgrCoolerTempOut
  EngOut29 : Outport  PortName=EngFdbk  Element=IntercoolerTempOut
  EngOut30 : Outport  PortName=EngFdbk  Element=BSFC
  EngOut31 : Outport  PortName=EngFdbk  Element=TPHC
  EngOut32 : Outport  PortName=EngFdbk  Element=TPCO
  EngOut33 : Outport  PortName=EngFdbk  Element=TPNOx
  EngOut34 : Outport  PortName=EngFdbk  Element=TPCO2
  EngOut35 : Outport  PortName=EngFdbk  Element=Iat
  EngOut36 : Outport  PortName=EngFdbk  Element=Ect
  EngOut37 : Outport  PortName=EngFdbk  Element=EgrVlvDeltaPrs
  EngOut38 : Outport  PortName=EngFdbk  Element=EgrVlvInTemp
  EngOut39 : Outport  PortName=EngFdbk  Element=CylPrs
  EngOut40 : Outport  PortName=EngFdbk  Element=EngTrqCrk
  EngOut41 : Outport  PortName=EngFdbk  Element=CrkAng
  wires:
  TPCO2/1 -> Signal Specification3/1
  ExhCamPhase/1 -> EngOut8/1
  IntkVlvLift/1 -> EngOut12/1
  CylPrs/1 -> Signal Specification4/1
  TurboSpd3/1 -> EngOut38/1
  IntkSwirlVlvPos/1 -> EngOut14/1
  TurboSpd2/1 -> EngOut29/1
  Bus Selector/6 -> EngOut19/1  "<ExhManGasTemp>"
  EngTrqCrk/1 -> Signal Specification6/1
  Map3/1 -> EngOut26/1
  Product/1 -> EngOut15/1
  Mat/1 -> EngOut4/1
  Bus Selector/1 -> Terminator3/1  "<EngSpd>"
  TurboSpd1/1 -> EngOut25/1
  Bus Selector/3 -> Product2/1  "<FuelVolFlw>"
  ClsdLpFuelMult/1 -> Product/2, Product1/2, Product2/2
  Map1/1 -> EngOut22/1
  EgrVlvAreaPct/1 -> EngOut10/1
  TurboRackPos/1 -> EngOut9/1
  Bus Selector/5 -> EngOut18/1  "<NrmlzdAirChrg>"
  Bus Selector/9 -> EngOut41/1  "<CrkAng>"
  VarIntkRunLen/1 -> EngOut13/1
  IntkCamPhase/1 -> EngOut7/1
  Bus Selector/2 -> Product/1  "<FuelMassFlw>"
  Mat3/1 -> EngOut37/1
  Bus Selector/4 -> EngOut17/1  "<IntkGasMassFlw>"
  Signal Specification1/1 -> EngOut32/1
  Product1/1 -> EngOut20/1
  WgAreaPct/1 -> EngOut6/1
  Map4/1 -> EngOut27/1
  VarCompRatioPos/1 -> EngOut11/1
  TurboSpd/1 -> EngOut21/1
  TPCO/1 -> Signal Specification1/1
  Signal Specification2/1 -> EngOut33/1
  Map2/1 -> EngOut23/1
  TPHC/1 -> Signal Specification5/1
  Mat2/1 -> EngOut28/1
  Map6/1 -> EngOut36/1
  Signal Specification3/1 -> EngOut34/1
  Signal Specification5/1 -> EngOut31/1
  ThrPosPct/1 -> EngOut5/1
  Map5/1 -> EngOut35/1
  Signal Specification6/1 -> EngOut40/1
  Map/1 -> EngOut3/1
  Bus Selector/8 -> EngOut30/1  "<Bsfc>"
  Signal Specification4/1 -> EngOut39/1
  Mat1/1 -> EngOut24/1
  Product2/1 -> EngOut16/1
  TPNOx/1 -> Signal Specification2/1
  FuelVolFlw/1 -> Bus Creator/5  "FuelVolFlw"
  ExhManGasTemp/1 -> Bus Creator/6  "ExhManGasTemp"
  EoCO/1 -> Bus Creator/12  "EoCO"
  IntkGasMassFlw/1 -> Bus Creator/1  "IntkGasMassFlw"
  PwrInfo/1 -> Bus Creator/16  "PwrInfo"
  EoCO2/1 -> Bus Creator/14  "EoCO2"
  EoPm/1 -> Bus Creator/15  "EoPm"
  FuelMassFlw/1 -> Bus Creator/4  "FuelMassFlw"
  CrkAng/1 -> Bus Creator/9  "CrkAng"
  Afr/1 -> Bus Creator/3  "Afr"
  EngSpd/1 -> EngOut2/1, Bus Creator/8  "EngSpd"
  EoNOx/1 -> Bus Creator/13  "EoNOx"
  NrmlzdAirChrg/1 -> Bus Creator/2  "NrmlzdAirChrg"
  Bsfc/1 -> Bus Creator/10  "Bsfc"
  EngTrq/1 -> Bus Creator/7, EngOut1/1  "EngTrq"
  Bus Creator/1 -> Bus Selector/1  "Info"
  EoHC/1 -> Bus Creator/11  "EoHC"
  Bus Selector/7 -> Product1/1  "<Afr>"

== system ConfiguredSimulinkPlantModels/Pedal, Cluster, Cabin/Brake Pedal ==
  DecelCmd : Inport
  Dead Zone1 : DeadZone  LowerValue=0  UpperValue=.01  ZeroCross=off
  DecelFdbk : Outport
  wires:
  Dead Zone1/1 -> DecelFdbk/1
  DecelCmd/1 -> Dead Zone1/1

== system ConfiguredSimulinkPlantModels/Sensors/Sensors ==
  VehFdbk : Inport
  No IMU Sensor : Subsystem  VariantControl=No IMU Sensor
  IMU : Outport

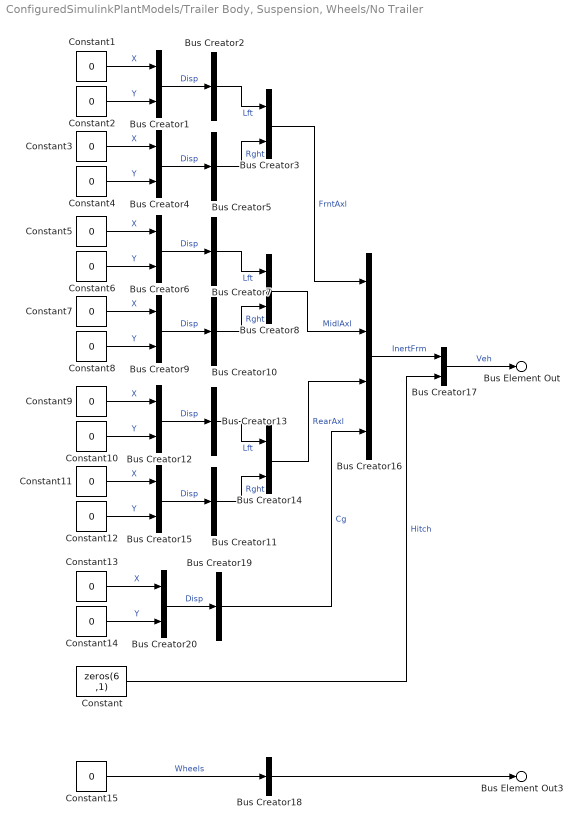
== system ConfiguredSimulinkPlantModels/Trailer Body, Suspension, Wheels/No Trailer ==
  Bus Creator{1,3..4,6,8..9,12,14..15,17,20} (11 alike) : BusCreator  Inputs=2
  Bus Creator{2,5,7,10..11,13,18..19} (8 alike) : BusCreator  Inputs=1
  Bus Creator16 : BusCreator  Inputs=4
  Constant : Constant  Value=zeros(6 ,1)  SampleTime=-1
  Constant{1..15} (15 alike) : Constant  Value=0  SampleTime=-1
  Bus Element Out3 : Outport  PortName=Wheels
  Bus Element Out : Outport  Port=2  PortName=Veh
  wires:
  Constant1/1 -> Bus Creator1/1  "X"
  Bus Creator18/1 -> Bus Element Out3/1
  Constant2/1 -> Bus Creator1/2  "Y"
  Bus Creator1/1 -> Bus Creator2/1  "Disp"
  Bus Creator4/1 -> Bus Creator5/1  "Disp"
  Constant4/1 -> Bus Creator4/2  "Y"
  Constant3/1 -> Bus Creator4/1  "X"
  Bus Creator5/1 -> Bus Creator3/2  "Rght"
  Bus Creator2/1 -> Bus Creator3/1  "Lft"
  Bus Creator7/1 -> Bus Creator8/1  "Lft"
  Bus Creator10/1 -> Bus Creator8/2  "Rght"
  Constant7/1 -> Bus Creator9/1  "X"
  Constant8/1 -> Bus Creator9/2  "Y"
  Bus Creator9/1 -> Bus Creator10/1  "Disp"
  Bus Creator6/1 -> Bus Creator7/1  "Disp"
  Constant6/1 -> Bus Creator6/2  "Y"
  Constant5/1 -> Bus Creator6/1  "X"
  Constant9/1 -> Bus Creator12/1  "X"
  Constant10/1 -> Bus Creator12/2  "Y"
  Bus Creator12/1 -> Bus Creator13/1  "Disp"
  Bus Creator15/1 -> Bus Creator11/1  "Disp"
  Constant12/1 -> Bus Creator15/2  "Y"
  Constant11/1 -> Bus Creator15/1  "X"
  Bus Creator11/1 -> Bus Creator14/2  "Rght"
  Bus Creator13/1 -> Bus Creator14/1  "Lft"
  Bus Creator8/1 -> Bus Creator16/2  "MidlAxl"
  Bus Creator14/1 -> Bus Creator16/3  "RearAxl"
  Bus Creator3/1 -> Bus Creator16/1  "FrntAxl"
  Bus Creator16/1 -> Bus Creator17/1  "InertFrm"
  Bus Creator17/1 -> Bus Element Out/1  "Veh"
  Constant15/1 -> Bus Creator18/1  "Wheels"
  Bus Creator19/1 -> Bus Creator16/4  "Cg"
  Constant13/1 -> Bus Creator20/1  "X"
  Constant14/1 -> Bus Creator20/2  "Y"
  Bus Creator20/1 -> Bus Creator19/1  "Disp"
  Constant/1 -> Bus Creator17/2  "Hitch"

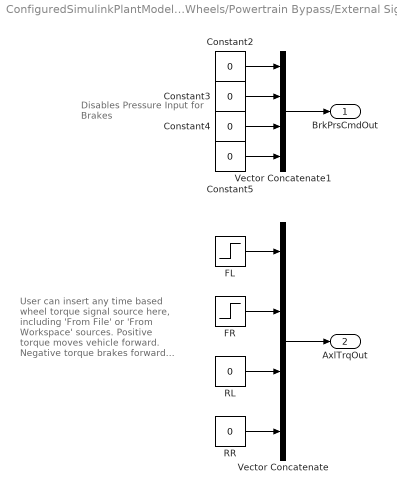
== system ConfiguredSimulinkPlantModels/Body, Suspension, Wheels/Powertrain Bypass/External Signal Source ==
  note: User can insert any time based
      | wheel torque signal source here,
      | including 'From File' or 'From
      | Workspace' sources.
      |
      | Positive torque moves vehicle
      | forward.
      | Negative torque brakes forward
      | moving vehicle or moves vehicle
      | in reverse.
  note: Disables Pressure
      | Input for Brakes
  Constant{2..5} (4 alike) : Constant  Value=0  SampleTime=-1
  FL : Step  After=100  SampleTime=0
  FR : Step  After=100  SampleTime=0
  RL : Constant  Value=0  SampleTime=-1
  RR : Constant  Value=0  SampleTime=-1
  Vector Concatenate : Concatenate  NumInputs=4
  Vector Concatenate1 : Concatenate  NumInputs=4
  BrkPrsCmdOut : Outport
  AxlTrqOut : Outport  Port=2
  wires:
  FL/1 -> Vector Concatenate/1
  FR/1 -> Vector Concatenate/2
  RL/1 -> Vector Concatenate/3
  RR/1 -> Vector Concatenate/4
  Vector Concatenate/1 -> AxlTrqOut/1
  Constant2/1 -> Vector Concatenate1/1
  Constant3/1 -> Vector Concatenate1/2
  Constant4/1 -> Vector Concatenate1/3
  Vector Concatenate1/1 -> BrkPrsCmdOut/1
  Constant5/1 -> Vector Concatenate1/4

== system ConfiguredSimulinkPlantModels/Body, Suspension, Wheels/Powertrain Bypass/Pass Through ==
  BrkPrsCmdIn : Inport
  AlxTrqIn : Inport  Port=2
  BrkPrsCmdOut : Outport
  AxlTrqOut : Outport  Port=2
  wires:
  AlxTrqIn/1 -> AxlTrqOut/1
  BrkPrsCmdIn/1 -> BrkPrsCmdOut/1

== system ConfiguredSimulinkPlantModels/Drivetrain/Drivetrain Layout/Axle Interconnect ==
  TrqSplitRatio : Inport
  SpdLock : Inport  Port=2
  FrntDiffrntlSpd : Inport  Port=3
  DriveshftTrq : Inport  Port=4
  RearDiffrntlSpd : Inport  Port=5
  No Interconnect : Subsystem  VariantControl=No Interconnect  ReferencedSubsystem=NoInterconnect
  DriveshftSpd : Outport
  FrntDiffrntlTrq : Outport  Port=2
  RearDiffrntlTrq : Outport  Port=3

== system ConfiguredSimulinkPlantModels/Drivetrain/Drivetrain Layout/DriveshftTrq Routing ==
  TrnsfrCaseFrntTrq : Inport
  DriveshftTrq : Inport  Port=2
  "TrnsfrCaseRearTrq " : Inport  Port=3
  One Actuator FWD : Subsystem  VariantControl=One Actuator FWD  ReferencedSubsystem=OneActuatorFWD
  FrntDiffrntlTrq : Outport
  TrnsfrCaseTrq : Outport  Port=2
  RearDiffrntlTrq : Outport  Port=3

== system ConfiguredSimulinkPlantModels/Drivetrain/Drivetrain Layout/Front Axle ==
  Prs1 : Inport
  Prs2 : Inport  Port=2
  DriveshftTrq : Inport  Port=3
  Axl1Trq : Inport  Port=4
  Axl2Trq : Inport  Port=5
  Open Differential : Subsystem  VariantControl=Open Differential  ReferencedSubsystem=OpenDifferential
  Info : Outport
  DriveshftSpd : Outport  Port=2
  Axl1Spd : Outport  Port=3
  Axl2Spd : Outport  Port=4

== system ConfiguredSimulinkPlantModels/Drivetrain/Drivetrain Layout/Front Axle Compliances ==
  RSpdL : Inport
  RSpdR : Inport  Port=2
  Omega : Inport  Port=3
  Axle Compliances : Subsystem  VariantControl=Axle Compliances  ReferencedSubsystem=AxleCompliances
  RTrqL : Outport
  RTrqR : Outport  Port=2
  CTrqL : Outport  Port=3
  CTrqR : Outport  Port=4

== system ConfiguredSimulinkPlantModels/Drivetrain/Drivetrain Layout/Rear Axle ==
  Prs1 : Inport
  Prs2 : Inport  Port=2
  DriveshftTrq : Inport  Port=3
  Axl1Trq : Inport  Port=4
  Axl2Trq : Inport  Port=5
  No Differential : Subsystem  VariantControl=No Differential  ReferencedSubsystem=NoDifferential
  Info : Outport
  DriveshftSpd : Outport  Port=2
  Axl1Spd : Outport  Port=3
  Axl2Spd : Outport  Port=4

== system ConfiguredSimulinkPlantModels/Drivetrain/Drivetrain Layout/Rear Axle Compliances ==
  Omega : Inport
  RSpdL : Inport  Port=2
  RSpdR : Inport  Port=3
  No Axle Compliances : Subsystem  VariantControl=No Axle Compliances  ReferencedSubsystem=NoAxleCompliances
  CTrqL : Outport
  CTrqR : Outport  Port=2
  RTrqL : Outport  Port=3
  RTrqR : Outport  Port=4

== system ConfiguredSimulinkPlantModels/Electrical System/Electrical System 1EM/Battery System ==
  note: 1) Add Subsystem or Model blocks as valid variant choices.
      | 2) You cannot connect blocks at this level. At simulation, connectivity is automatically
      | determined, based on the active variant and port name matching.
  LdCurr : Inport
  BattTemp : Inport  Port=2
  Mapped Battery : Subsystem  VariantControl=Mapped Battery  ReferencedSubsystem=Battery
  BattSoc : Outport  VectorParamsAs1DForOutWhenUnconnected=off
  BattCurr : Outport  Port=2  VectorParamsAs1DForOutWhenUnconnected=off
  BattVolt : Outport  Port=3  VectorParamsAs1DForOutWhenUnconnected=off
  BMSSensors : Outport  Port=4  VectorParamsAs1DForOutWhenUnconnected=off

== system ConfiguredSimulinkPlantModels/Electrical System/Electrical System 1EM/DC-DC Converter ==
  BatVolt : Inport
  LdCurr : Inport  Port=2
  VoltCmd : Inport  Port=3
  No DC-DC Converter : Subsystem  VariantControl=No DC-DC Converter  ReferencedSubsystem=NoDCDCConverter
  BusVolt : Outport
  SrcCurr : Outport  Port=2

== system ConfiguredSimulinkPlantModels/Electrical System/Electrical System 1EM/Electric Machine 1 ==
  EMTrqCmd : Inport
  EMSpd : Inport  Port=2
  BusVolt : Inport  Port=3
  Mapped EM : Subsystem  VariantControl=Mapped EM  ReferencedSubsystem=ElectricMachine1
  EMTrq : Outport  VectorParamsAs1DForOutWhenUnconnected=off
  EMCurr : Outport  Port=2  VectorParamsAs1DForOutWhenUnconnected=off
  EMPwrMech : Outport  Port=3

== system ConfiguredSimulinkPlantModels/Sensors/Sensors/No IMU Sensor ==
  VehFdbk : Inport
  Bus Creator1 : BusCreator  Inputs=2
  Constant : Constant  Value=zeros(3,1)  SampleTime=-1
  Constant1 : Constant  Value=zeros(3,1)  SampleTime=-1
  Terminator : Terminator
  IMU : Outport
  wires:
  VehFdbk/1 -> Terminator/1
  Constant1/1 -> Bus Creator1/2  "pqr"
  Bus Creator1/1 -> IMU/1  "IMU"
  Constant/1 -> Bus Creator1/1  "Acc"
